simulink model "IRlineFollowInitialVersion"  (R2023b)
settings: Solver=FixedStepAuto  StartTime=0.0  StopTime=inf  RelTol=1e-3  EnableMultiTasking=on
libraries: vexarmcortexlib x5
settings Model: Creator=ierdn  LastModifiedBy=ierdn
settings DataIOCC: LimitDataPoints=on  SignalLoggingSaveFormat=ModelDataLogs  ReturnWorkspaceOutputs=off
settings OptimizationCC: ExpressionDepthLimit=2147483647  LifeSpan=Inf  MaxStackSize=64  EfficientTunableParamExpr=on
settings DebuggingCC: UnderspecifiedInitializationDetection=Classic  MergeDetectMultiDrivingBlocksExec=none  InheritedTsInSrcMsg=none  FcnCallInpInsideContextMsg=warning  StateNameClashWarn=warning  SFUnexpectedBacktrackingDiag=warning  SFNoUnconditionalDefaultTransitionDiag=warning  SFExecutionAtInitializationDiag=none  ArithmeticOperatorsInVariantConditions=warning
settings HardwareCC: ProdBitPerPointer=32  ProdBitPerSizeT=32  ProdBitPerPtrDiffT=32  ProdLargestAtomicInteger=Long  ProdLargestAtomicFloat=Double  ProdIntDivRoundTo=Undefined  ProdWordSize=32  ProdHWDeviceType=ARM Compatible->ARM Cortex
settings ModelReferenceCC: EnableRefExpFcnMdlSchedulingChecks=on  PropagateSignalLabelsOutOfModel=off
settings SFSimCC: MATLABDynamicMemAlloc=off  CustomCodeUndefinedFunction=UseInterfaceOnly
settings RTWCC: Description=Embedded Coder  SystemTargetFile=ert.tlc  HardwareBoard=ARM Cortex-based VEX Microcontroller  TemplateMakefile=ert_default_tmf  Toolchain=GNU Tools for VEX ARM Cortex
settings CodeAppCC: IgnoreCustomStorageClasses=off  CustomSymbolStrType=$N$R$M  StateflowObjectComments=on  InternalIdentifier=Classic
settings ERTTargetCC: CodeReplacementLibrary=GCC ARM Cortex-M3  MultiwordLength=2048  ConvertIfToSwitch=off  SuppressUnreachableDefaultCases=off

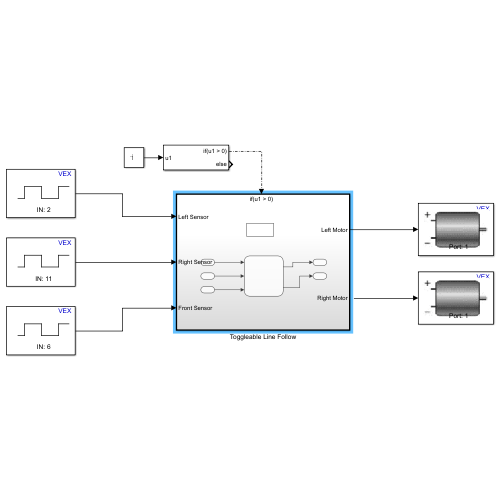
[thumbnail: Simulink's stored preview of the top-level diagram]
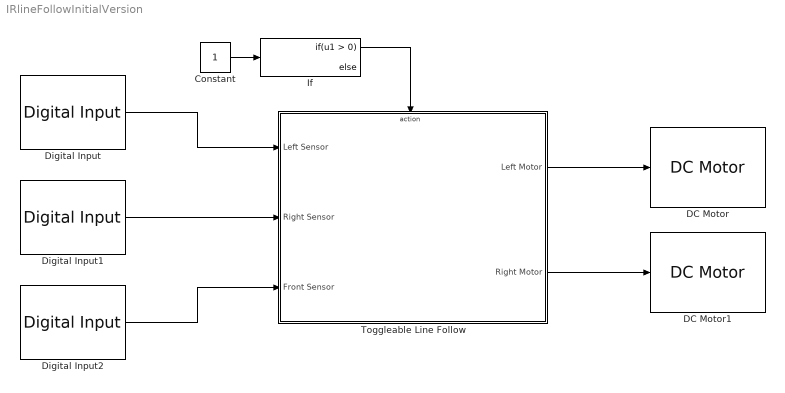
== system IRlineFollowInitialVersion ==
  Constant : Constant
  DC Motor : vexarmcortexlib/Actuators/DC Motor  motor=1  scaleFactor=1/13.5  SimulationOut=off
  DC Motor1 : vexarmcortexlib/Actuators/DC Motor  motor=1  scaleFactor=1/13.5  SimulationOut=off
  Digital Input : vexarmcortexlib/Sensors/Digital Input  inChan=2  SimulationIn=off  SampleTime=0.2
  Digital Input1 : vexarmcortexlib/Sensors/Digital Input  inChan=11  SimulationIn=off  SampleTime=0.2
  Digital Input2 : vexarmcortexlib/Sensors/Digital Input  inChan=6  SimulationIn=off  SampleTime=0.2
  If : If
  Toggleable Line Follow : Subsystem  TreatAsAtomicUnit=on
  wires:
  Constant/1 -> If/1
  If/1 -> Toggleable Line Follow/Action
  Digital Input/1 -> Toggleable Line Follow/1(Left Sensor)
  Digital Input1/1 -> Toggleable Line Follow/2(Right Sensor)
  Digital Input2/1 -> Toggleable Line Follow/3(Front Sensor)
  Toggleable Line Follow/1(Left Motor) -> DC Motor/1
  Toggleable Line Follow/2(Right Motor) -> DC Motor1/1

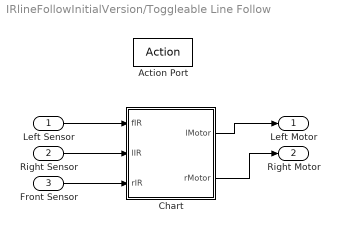
== system IRlineFollowInitialVersion/Toggleable Line Follow ==
  Left Sensor : Inport
  Right Sensor : Inport  Port=2
  Front Sensor : Inport  Port=3
  Action Port : ActionPort  ActionPortLabel=if(u1 > 0)
  Chart : Stateflow chart  TreatAsAtomicUnit=on
  Left Motor : Outport
  Right Motor : Outport  Port=2
  wires:
  Left Sensor/1 -> Chart/1(fIR)
  Chart/1(lMotor) -> Left Motor/1
  Chart/2(rMotor) -> Right Motor/1
  Right Sensor/1 -> Chart/2(lIR)
  Front Sensor/1 -> Chart/3(rIR)

== stateflow chart IRlineFollowInitialVersion/Toggleable Line Follow/Chart ==
  state Start
    fin = 0;
    brainDetect = 0;
  state forwardLine
    Forward;
  state backwardLine
    Backward;
  state Stop
    fin = 0;
  (default) -> Start
  Start -> (junction 25)
  (junction 25) -> forwardLine [order 1] : [fin == 0 && brainDetect == 0]
  (junction 25) -> backwardLine [order 3] : [fin == 0 &&  brainDetect ==1]
      | {lMotor =  -50; rMotor = -50;}
  backwardLine -> (junction 25) : [fin == 1]
  forwardLine -> (junction 25) : [brainDetect == 1]
  (junction 25) -> Stop [order 2] : [fin == 1]
  data: fIR input; lIR input; rIR input; lMotor output [-127..127] =50; rMotor output [-127..127] =50; fin local; brainDetect local [0..1] =0
  function Forward:
    | function Forward
    | 
    | init();
    | 
    | lIREQ0 = false;
    | rIREQ0 = false;
    | fIREQ0 = false;
    | 
    | 
    | % Left IR is equal to 0
    | 
    | lIREQ0 = logical(lIR == 0);
    | 
    | % Right IR is equal to 0
    | 
    | rIREQ0 = logical(rIR == 0);
    | 
    | % Front IR is equal to 0
    | 
    | fIREQ0 = logical(fIR == 0);
    | 
    | if (~lIREQ0 && rIREQ0 && ~fIREQ0)
    |     A4();
    | elseif (lIREQ0 && ~rIREQ0 && ~fIREQ0)
    |     A1();
    | elseif (lIREQ0 && rIREQ0 && ~fIREQ0)
    |     A1();
    | elseif (~lIREQ0 && ~rIREQ0 && ~fIREQ0)
    |     A2();
    | elseif (~lIREQ0 && ~rIREQ0 && fIREQ0)
    |     A3();
    | elseif (lIREQ0 && ~rIREQ0 && fIREQ0)
    |     A3();
    | elseif (lIREQ0 && rIREQ0 && fIREQ0)
    |     A3();
    | else % Default
    |     A3();
    | end
    | 
    | final();
    | 
    | function init()
    | 
    | % Initial
    | 
    | coder.extrinsic("disp");
    | 
    | disp("truth table ttable entered");
    | 
    | function A1()
    | 
    | % Left IR is seeing white - turn Left
    | 
    | lMotor == lMotor/1.5;
    | 
    | function A2()
    | 
    | % Right IR is seeing black - turn Right
    | 
    | rMotor == rMotor/1.5;
    | 
    | function A3()
    | 
    | % fIR is seeing the brain and the sensors are alighned - Stop
    | 
    | rMotor == 0 && lMotor == 0 &&brainDetect == 1;
    | 
    | function A4()
    | 
    | % Everything is good
    | 
    | rMotor == 50 && rMotor == 50;
    | 
    | function final()
    | 
    | % Final
    | 
    | coder.extrinsic("disp");
    | 
    | disp("truth table ttable exited");
  function Backward:
    | function Backward
    | 
    | init();
    | 
    | lIREQ0 = false;
    | rIREQ0 = false;
    | fIREQ0 = false;
    | 
    | 
    | % Left IR is equal to 0
    | 
    | lIREQ0 = logical(lIR == 0);
    | 
    | % Right IR is equal to 0
    | 
    | rIREQ0 = logical(rIR == 0);
    | 
    | % Front IR is equal to 0
    | 
    | fIREQ0 = logical(fIR == 0);
    | 
    | if (~lIREQ0 && rIREQ0 && ~fIREQ0)
    |     A4();
    | elseif (lIREQ0 && ~rIREQ0 && ~fIREQ0)
    |     A1();
    | elseif (lIREQ0 && rIREQ0 && ~fIREQ0)
    |     A1();
    | elseif (~lIREQ0 && ~rIREQ0 && ~fIREQ0)
    |     A2();
    | elseif (~lIREQ0 && ~rIREQ0 && fIREQ0)
    |     A3();
    | elseif (lIREQ0 && ~rIREQ0 && fIREQ0)
    |     A3();
    | elseif (lIREQ0 && rIREQ0 && fIREQ0)
    |     A3();
    | else % Default
    |     A3();
    | end
    | 
    | final();
    | 
    | function init()
    | 
    | % Initial
    | 
    | coder.extrinsic("disp");
    | 
    | disp("truth table ttable entered");
    | 
    | function A1()
    | 
    | % Left IR is seeing white - turn Left
    | 
    | lMotor == lMotor/1.5;
    | 
    | function A2()
    | 
    | % Right IR is seeing black - turn Right
    | 
    | rMotor == rMotor/1.5;
    | 
    | function A3()
    | 
    | % fIR is seeing the brain and the sensors are alighned - Stop
    | 
    | rMotor == 0 && lMotor == 0 && fin == 1;
    | 
    | function A4()
    | 
    | % Everything is good
    | 
    | rMotor == 50 && rMotor == 50;
    | 
    | function final()
    | 
    | % Final
    | 
    | coder.extrinsic("disp");
    | 
    | disp("truth table ttable exited");
